simulink model "simulation"  (Simulink 8.9)
settings: Solver=ode4  StartTime=0.0  StopTime=2.0  MaxStep=1e-4  RelTol=1e-3
undefined symbols (not defined in the file): Hydride, Metal, Nickel
libraries: powerlib x12, simulink x2, electricdrivelib x1, powerlib_meascontrol x1
settings Model: Creator=HemanthSai  LastModifiedBy=HemanthSai
settings DataIOCC: LimitDataPoints=off  SaveFormat=Dataset  SignalLoggingSaveFormat=Dataset
settings OptimizationCC: LifeSpan=auto
settings DebuggingCC: UnderspecifiedInitializationDetection=Simplified  MergeDetectMultiDrivingBlocksExec=error  FcnCallInpInsideContextMsg=error  UnconnectedInputMsg=none  UnconnectedOutputMsg=none  UnconnectedLineMsg=none  StateNameClashWarn=none  SFUnexpectedBacktrackingDiag=error  SFNoUnconditionalDefaultTransitionDiag=error  SFExecutionAtInitializationDiag=warning
settings HardwareCC: ProdBitPerPointer=64  ProdBitPerSizeT=64  ProdBitPerPtrDiffT=64  ProdLargestAtomicFloat=Float  ProdIntDivRoundTo=Zero  ProdEndianess=LittleEndian  ProdWordSize=64  ProdHWDeviceType=Intel->x86-64 (Windows64)
settings ModelReferenceCC: PropagateSignalLabelsOutOfModel=on
settings GRTTargetCC: TargetLangStandard=C99 (ISO)  GeneratePreprocessorConditionals=Use local settings  CombineOutputUpdateFcns=on  GRTInterface=off
settings ConfigComp: CovMetricSettings=dwe  CovHtmlReporting=off  CovSaveCumulativeToWorkspaceVar=off  CovSaveSingleToWorkspaceVar=off  CovExternalEMLEnable=on

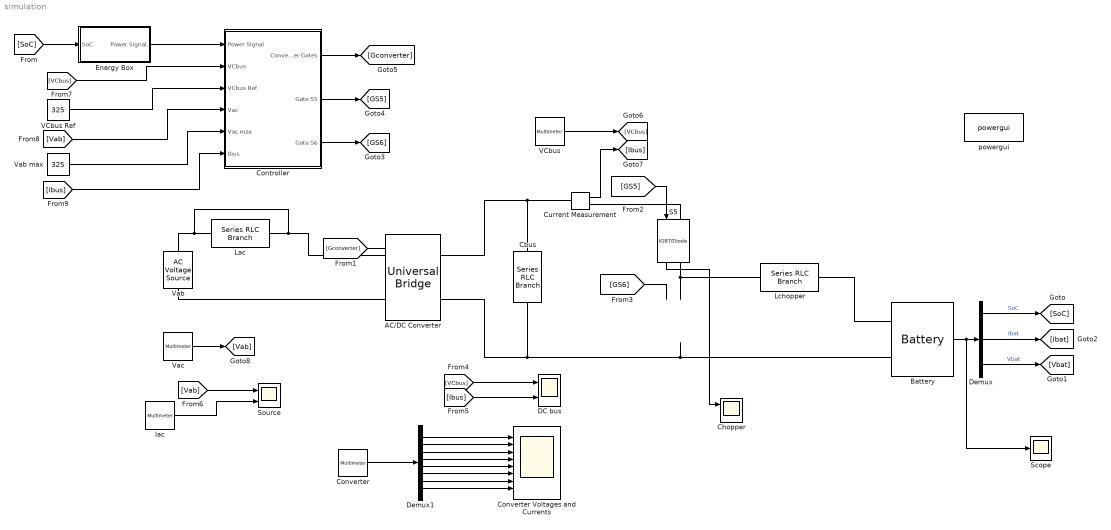
== system simulation ==
  AC/DC Converter : powerlib/Power Electronics/Universal Bridge  Arms=2  SnubberResistance=1e5  SnubberCapacitance=inf  Device=Diodes  Ron=1e-3  Lon=0  ForwardVoltages="[  0  0  ]"  ForwardVoltage=0  GTOparameters=[ 10e-6 , 20e-6 ]  IGBTparameters=[ 1e-6 , 2e-6 ]  Measurements=All voltages and currents  Measurements_2=None  converterType=Rectifier
  Battery : electricdrivelib/Extra Sources/Battery  BatType=Nickel-Metal-Hydride  ShowTempParam=off  ThermalPreset=no  ShowAgeParam=off  NomV=96  NomQ=100  SOC=50  Batt_Tr=1  PresetModel=on  MaxQ=107.6923  MinV=72  FullV=113.0847  Dis_rate=20  R=0.0096  Normal_OP=96.1538  expZone="[104.1356            20]"  current=[6.5 13 32.5]  Units=Ampere-hour  Tci=20  NomT=20  T2=-30  MaxQ2=4.8  FullV2=7.1  Normal_OP2=5.655  expZone2="[6.58           1]"  Rca=0.6  ti=2000  Dp=0  Neq0=0  Tsim=1e6  Ta1=25  Qeol=5.4*0.9  Reol=0.013333*1.2  Char_age=[2.3478, 3]  Dis_age=[2.3478, 10]  N1=1500  N2=10500  N3=1000  N4=1400  Ta2=45  N5=950
  Cbus : powerlib/Elements/Series RLC Branch  LConnTagsString=__new0  RConnTagsString=__new0  BranchType=C  Resistance=1  Inductance=1e-3  SetiL0=off  InitialCurrent=0  Capacitance=10e-3  Setx0=off  InitialVoltage=0  Measurements=Branch voltage
  Chopper : Scope  NumInputPorts=2
  Controller : Subsystem
  Converter : powerlib/Measurements/Multimeter  PhasorSimulation=off  OutputType=Complex  sel=[2 3 4 5 9 10 11 12]  L=12  Gain=[1 1 1 1 1 1 1 1]  yselected={'Usw1: AC//DC Converter','Usw2: AC//DC Converter','Usw3: AC//DC Converter','Usw4: AC//DC Converter','Isw1: AC//DC Converter','Isw2: AC//DC Converter','Isw3: AC//DC Converter','Isw4: AC//DC Converter'};  PSBOutputType=1  PSBequivalent=0  AxesSetting=[0,0.1,-100,100]  Display=0  SavedBlockNames=-11
  Converter Voltages and Currents : Scope  NumInputPorts=8
  Current Measurement : powerlib/Measurements/Current Measurement  PhasorSimulation=off  OutputType=Complex  PSBequivalent=0
  DC bus : Scope  NumInputPorts=2
  Demux : Demux  Outputs=3
  Demux1 : Demux  Outputs=8
  Energy Box : Subsystem
  Iac : powerlib/Measurements/Multimeter  PhasorSimulation=off  OutputType=Complex  sel=1  L=12  Gain=0  yselected={}  PSBOutputType=1  PSBequivalent=0  AxesSetting=[0,0.1,-100,100]  Display=0  SavedBlockNames=-11
  Lac : powerlib/Elements/Series RLC Branch  LConnTagsString=__new0  RConnTagsString=__new0  BranchType=L  Resistance=1  Inductance=7.6e-3  SetiL0=off  InitialCurrent=0  Capacitance=1e-6  Setx0=off  InitialVoltage=0  Measurements=Branch current
  Lchopper : powerlib/Elements/Series RLC Branch  LConnTagsString=__new0  RConnTagsString=__new0  BranchType=L  Resistance=1  Inductance=1.9e-3  SetiL0=off  InitialCurrent=0  Capacitance=1e-6  Setx0=off  InitialVoltage=0  Measurements=None
  S5 : powerlib/Power Electronics/IGBT//Diode  Ron=1e-3  Rs=1e5  Cs=inf  Measurements=on
  Scope : Scope
  Source : Scope  NumInputPorts=2
  VCbus : powerlib/Measurements/Multimeter  PhasorSimulation=off  OutputType=Complex  sel=1  L=12  Gain=1  yselected={'Ub: Cbus'};  PSBOutputType=1  PSBequivalent=0  AxesSetting=[0,0.1,-100,100]  Display=0  SavedBlockNames=-11
  VCbus Ref : Constant  Value=325
  Vab : powerlib/Electrical Sources/AC Voltage Source  Amplitude=325  Phase=0  Frequency=50  SampleTime=0  Measurements=Voltage  BusType=swing  Pref=10e3  Qref=0  Qmin=-inf  Qmax=+inf
  Vab max : Constant  Value=325
  Vac : powerlib/Measurements/Multimeter  PhasorSimulation=off  OutputType=Complex  sel=8  L=12  Gain=1  yselected={'Usrc: Vab'};  PSBOutputType=1  PSBequivalent=0  AxesSetting=[0,0.1,-100,100]  Display=0  SavedBlockNames=-11
  powergui : powerlib/powergui  Priority=1  SimulationMode=Discrete  SampleTime=50e-6  frequency=60  Iterations=50  frequencyindice=50  Pbase=100e6  ErrMax=1e-4  UnitsV=kV  UnitsW=MW  buscounter=0  FunctionMessages=off  echomessages=off  EnableUseOfTLC=off  CurrentSourceSwitches=off  DisableSnubberDevices=off  DisableRonSwitches=off  DisableVfSwitches=off  DisplayEquations=off  SolverType=Tustin/Backward Euler (TBE)  Interpol=off  ExternalGateDelay=off  methode=off  Ts=100  x0status=blocks  SPID=on  SwTol=0  HookPort=off  RestoreLinks=warning  ResistiveCurrentMeasurement=off  Frange=[0:2:500]  Ylog=off  Xlog=on  ShowGrid=off  save=off  variable=ZData  structure=0  ZoomFFT=off  StartTime=0.0  cycles=1  DisplayStyle=1  fundamental=60  FreqAxis=off  MaxFrequency=1000  frequencyindicesteady=1  RmsSteady=1  display=off
  wires:
  Battery/1 -> Scope/1, Demux/1
  VCbus/1 -> [VCbus]
  Demux/1 -> [SoC]  "SoC"
  Demux/2 -> [Ibat]  "Ibat"
  Demux/3 -> [Vbat]  "Vbat"
  S5/1 -> Chopper/1
  ? -> Chopper/2
  Iac/1 -> Source/2
  Current Measurement/1 -> [Ibus]
  [SoC] -> Energy Box/1(SoC)
  Energy Box/1(Power Signal) -> Controller/1(Power Signal)
  Converter/1 -> Demux1/1
  Demux1/1 -> Converter Voltages and Currents/1
  Demux1/2 -> Converter Voltages and Currents/2
  Demux1/3 -> Converter Voltages and Currents/3
  Demux1/4 -> Converter Voltages and Currents/4
  Demux1/5 -> Converter Voltages and Currents/5
  Demux1/6 -> Converter Voltages and Currents/6
  Demux1/7 -> Converter Voltages and Currents/7
  Demux1/8 -> Converter Voltages and Currents/8
  Controller/1(Converter Gates) -> [Gconverter]
  Controller/2(Gate S5) -> [GS5]
  Controller/3(Gate S6) -> [GS6]
  [Gconverter] -> ?
  [GS5] -> S5/1
  [GS6] -> ?
  [VCbus] -> DC bus/1
  [Ibus] -> DC bus/2
  Vac/1 -> [Vab]
  [Vab] -> Source/1
  VCbus Ref/1 -> Controller/3(VCbus Ref)
  [VCbus] -> Controller/2(VCbus)
  [Vab] -> Controller/4(Vac)
  Vab max/1 -> Controller/5(Vac max)
  [Ibus] -> Controller/6(Ibus)
  connections:
  Lac/RConn1 -- Lac/LConn1 -- Vab/RConn1 -- AC/DC Converter/LConn1
  Lchopper/LConn1 -- S5/RConn1
  Cbus/LConn1 -- Current Measurement/LConn1 -- AC/DC Converter/RConn1
  Vab/LConn1 -- AC/DC Converter/LConn2
  Lchopper/RConn1 -- Battery/LConn1
  Current Measurement/RConn1 -- S5/LConn1
  Battery/LConn2 -- Cbus/RConn1 -- AC/DC Converter/RConn2

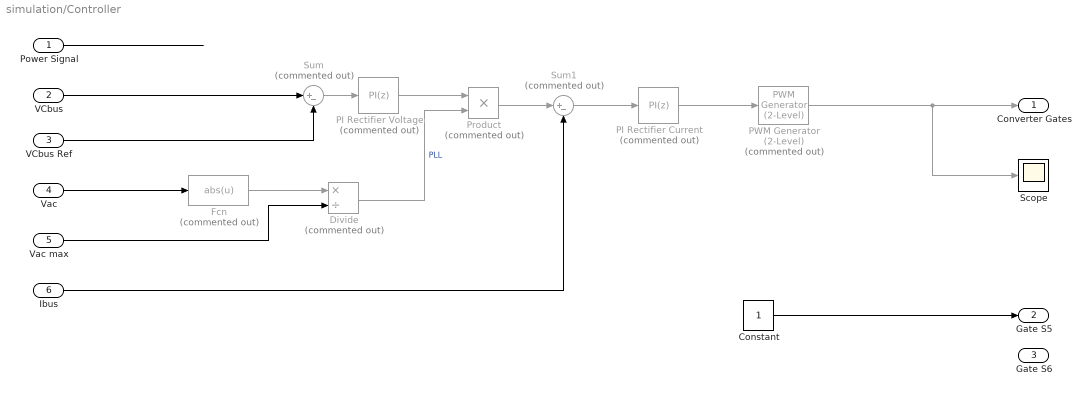
== system simulation/Controller ==
  Power Signal : Inport
  VCbus : Inport  Port=2
  VCbus Ref : Inport  Port=3
  Vac : Inport  Port=4
  Vac max : Inport  Port=5
  Ibus : Inport  Port=6
  Constant : Constant
  Divide : Product  Commented=on  Inputs=*/
  Fcn : Fcn  Commented=on  Expr=abs(u)
  PI Rectifier Current : simulink/Continuous/PID Controller  Commented=on  Controller=PI  TimeDomain=Discrete-time  SampleTime=-1  IntegratorMethod=Forward Euler  FilterMethod=Forward Euler  Form=Parallel  UseFilter=on  ControllerParametersSource=internal  P=5.2  I=1.3  D=0  N=100  InitialConditionSource=internal  InitialConditionForIntegrator=0  InitialConditionForFilter=0  ExternalReset=none  LimitOutput=off  UpperSaturationLimit=inf  LowerSaturationLimit=-inf  LinearizeAsGain=on  AntiWindupMode=none  Kb=1  TrackingMode=off  Kt=1  PParamMin=[]  PParamMax=[]  IParamMin=[]  IParamMax=[]  DParamMin=[]  DParamMax=[]  NParamMin=[]  NParamMax=[]  KbParamMin=[]  KbParamMax=[]  KtParamMin=[]  KtParamMax=[]  POutMin=[]  POutMax=[]  IOutMin=[]  IOutMax=[]  DOutMin=[]  DOutMax=[]  NOutMin=[]  NOutMax=[]  KbOutMin=[]  KbOutMax=[]  KtOutMin=[]  KtOutMax=[]  IntegratorOutMin=[]  IntegratorOutMax=[]  FilterOutMin=[]  FilterOutMax=[]  SumOutMin=[]  SumOutMax=[]  SumI1OutMin=[]  SumI1OutMax=[]  SumI2OutMin=[]  SumI2OutMax=[]  SumI3OutMin=[]  SumI3OutMax=[]  SumDOutMin=[]  SumDOutMax=[]  SaturationOutMin=[]  SaturationOutMax=[]  IntegratorContinuousStateAttributes=''  IntegratorStateMustResolveToSignalObject=off  IntegratorRTWStateStorageClass=Auto  FilterContinuousStateAttributes=''  FilterStateMustResolveToSignalObject=off  FilterRTWStateStorageClass=Auto  DifferentiatorICPrevScaledInput=0  DifferentiatorOutMin=[]  DifferentiatorOutMax=[]  InitialConditionSetting=State (most efficient)
  PI Rectifier Voltage : simulink/Continuous/PID Controller  Commented=on  Controller=PI  TimeDomain=Discrete-time  SampleTime=-1  IntegratorMethod=Forward Euler  FilterMethod=Forward Euler  Form=Parallel  UseFilter=on  ControllerParametersSource=internal  P=11.7  I=0.87  D=0  N=100  InitialConditionSource=internal  InitialConditionForIntegrator=0  InitialConditionForFilter=0  ExternalReset=none  LimitOutput=off  UpperSaturationLimit=inf  LowerSaturationLimit=-inf  LinearizeAsGain=on  AntiWindupMode=none  Kb=1  TrackingMode=off  Kt=1  PParamMin=[]  PParamMax=[]  IParamMin=[]  IParamMax=[]  DParamMin=[]  DParamMax=[]  NParamMin=[]  NParamMax=[]  KbParamMin=[]  KbParamMax=[]  KtParamMin=[]  KtParamMax=[]  POutMin=[]  POutMax=[]  IOutMin=[]  IOutMax=[]  DOutMin=[]  DOutMax=[]  NOutMin=[]  NOutMax=[]  KbOutMin=[]  KbOutMax=[]  KtOutMin=[]  KtOutMax=[]  IntegratorOutMin=[]  IntegratorOutMax=[]  FilterOutMin=[]  FilterOutMax=[]  SumOutMin=[]  SumOutMax=[]  SumI1OutMin=[]  SumI1OutMax=[]  SumI2OutMin=[]  SumI2OutMax=[]  SumI3OutMin=[]  SumI3OutMax=[]  SumDOutMin=[]  SumDOutMax=[]  SaturationOutMin=[]  SaturationOutMax=[]  IntegratorContinuousStateAttributes=''  IntegratorStateMustResolveToSignalObject=off  IntegratorRTWStateStorageClass=Auto  FilterContinuousStateAttributes=''  FilterStateMustResolveToSignalObject=off  FilterRTWStateStorageClass=Auto  DifferentiatorICPrevScaledInput=0  DifferentiatorOutMin=[]  DifferentiatorOutMax=[]  InitialConditionSetting=State (most efficient)
  PWM Generator (2-Level) : powerlib_meascontrol/Pulse & Signal Generators/PWM Generator (2-Level)  Commented=on  ModulatorType=Single-phase full-bridge (4 pulses)  ModulatorMode=Unsynchronized  Fc=27*60  Pc=90  nF=27  MinMax="[ -1  1 ]"  SamplingTechnique=Natural  ModulatingSignals=off  m=0.8  Freq=60  Phase=0  Ts=0  ShowCarrierOutport=off
      settings: SourceProductName=Simscape Power Systems
  Product : Product  Commented=on
  Scope : Scope
  Sum : Sum  Commented=on  Inputs=|+-
  Sum1 : Sum  Commented=on  Inputs=|+-
  Converter Gates : Outport
  Gate S5 : Outport  Port=2
  Gate S6 : Outport  Port=3
  wires:
  Power Signal/1 -> ?
  VCbus/1 -> Sum/1
  VCbus Ref/1 -> Sum/2
  Vac/1 -> Fcn/1
  Fcn/1 -> Divide/1
  Vac max/1 -> Divide/2
  Divide/1 -> Product/2  "PLL"
  Sum/1 -> PI Rectifier Voltage/1
  PI Rectifier Voltage/1 -> Product/1
  Ibus/1 -> Sum1/2
  Product/1 -> Sum1/1
  Sum1/1 -> PI Rectifier Current/1
  PI Rectifier Current/1 -> PWM Generator (2-Level)/1
  PWM Generator (2-Level)/1 -> Scope/1, Converter Gates/1
  Constant/1 -> Gate S5/1

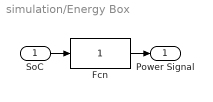
== system simulation/Energy Box ==
  SoC : Inport
  Fcn : Fcn  Expr=1
  Power Signal : Outport
  wires:
  SoC/1 -> Fcn/1
  Fcn/1 -> Power Signal/1
